simulink model "calculations"  (R2014b)
settings: Solver=ode45  StartTime=0.0  StopTime=10.0  RelTol=1e-3
values from neighbouring files (symbols this model uses):
  A = [0 1 0 0 ... (first row only)    [calculations.m]
  B = [0 ... (first row only)    [calculations.m]
  C = [1 0 0 0 ... (first row only)    [calculations.m]
  D = [0 ... (first row only)    [calculations.m]
  K = lqr(sys,Q,R)    [calculations.m]
settings Model: Creator=samsung  LastModifiedBy=Stahu
settings DebuggingCC: UnderspecifiedInitializationDetection=Classic  MergeDetectMultiDrivingBlocksExec=none  StateNameClashWarn=warning

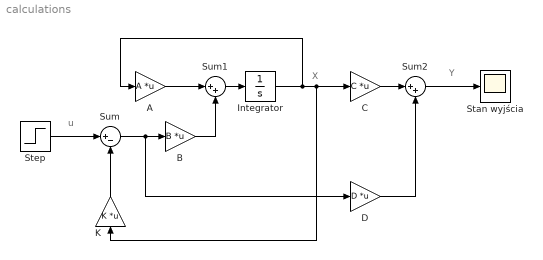
== system calculations ==
  note: Y
  note: X
  note: u
  A : Gain  Gain=A  Multiplication=Matrix(K*u)
  B : Gain  Gain=B  Multiplication=Matrix(K*u)
  C : Gain  Gain=C  Multiplication=Matrix(K*u)
  D : Gain  Gain=D  Multiplication=Matrix(K*u)
  Integrator : Integrator
  K : Gain  Gain=K  Multiplication=Matrix(K*u)
  Stan wyjścia : Scope
  Step : Step  Time=0  SampleTime=0
  Sum : Sum  Inputs=|+-
  Sum1 : Sum  Inputs=|++
  Sum2 : Sum  Inputs=|++
  wires:
  Step/1 -> Sum/1
  B/1 -> Sum1/2
  A/1 -> Sum1/1
  Sum1/1 -> Integrator/1
  C/1 -> Sum2/1
  D/1 -> Sum2/2
  Integrator/1 -> A/1, K/1, C/1
  Sum2/1 -> Stan wyjścia/1
  Sum/1 -> D/1, B/1
  K/1 -> Sum/2
